simulink model "fivestatespace_revised"  (R2020a)
settings: Solver=VariableStepAuto  StartTime=0.0  StopTime=10.00  RelTol=1e-3
values from neighbouring files (symbols this model uses):
  alpha = (slope*pi)/180    (= 0)    [milestone2constants.m]
  Beq = 0.2963    [milestone2constants.m]
  Fd = 0    [milestone2constants.m]
  Jeq = 0.01802    [milestone2constants.m]
  Kb = 2.2179e-3    (= 0.0022179)    [milestone2constants.m]
  Keq = 0.74    [milestone2constants.m]
  Mg = M*g    (= 15.5979)    [milestone2constants.m]
  Mgmu = M*g*mu    (= 0)    [milestone2constants.m]
  r = 0.037    [milestone2constants.m]
  ra = 7.4    [milestone2constants.m]
  step_time = 10    [milestone2constants.m]
  theta_i = 0    [milestone2constants.m]
  threshold = 5    [milestone2constants.m]
  u_l_f = 9    [milestone2constants.m]
  u_l_i = 10    [milestone2constants.m]
  u_r_f = 3    [milestone2constants.m]
  u_r_i = 5    [milestone2constants.m]
  v_i = 0    [milestone2constants.m]
  v_txy = 0    [milestone2constants.m]
  v_w = 0    [milestone2constants.m]
  wl_i = 0    [milestone2constants.m]
  Wr = 0.18    [milestone2constants.m]
  wr_i = 0    [milestone2constants.m]
  x_i = 0    [milestone2constants.m]
  y_i = 0    [milestone2constants.m]
undefined symbols (not defined in the file or in its folder): k
settings Model: Creator=oliviaball  LastModifiedBy=oliviaball
settings DataIOCC: ReturnWorkspaceOutputs=off
settings DebuggingCC: ArithmeticOperatorsInVariantConditions=warning
settings SFSimCC: CustomCodeUndefinedFunction=UseInterfaceOnly

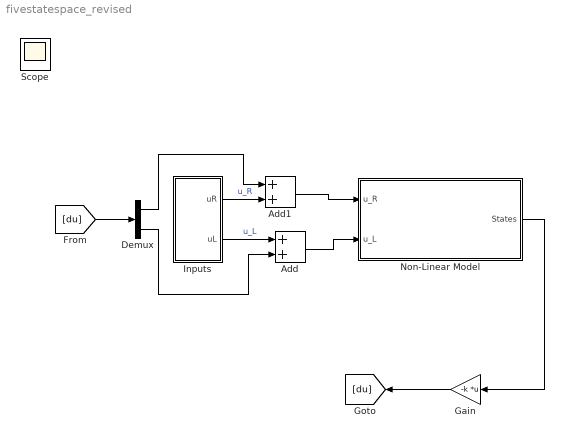
== system fivestatespace_revised ==
  Add : Sum
  Add1 : Sum
  Demux : Demux  Outputs=2
  Gain : Gain  Gain=-k  Multiplication=Matrix(K*u)
  Inputs : Subsystem
  Non-Linear Model : Subsystem
  Scope : Scope
  wires:
  Non-Linear Model/1(States) -> Gain/1
  Gain/1 -> [du]
  [du] -> Demux/1
  Inputs/2(uL) -> Add/1  "u_L"
  Add/1 -> Non-Linear Model/2(u_L)
  Demux/2 -> Add/2
  Inputs/1(uR) -> Add1/2  "u_R"
  Add1/1 -> Non-Linear Model/1(u_R)
  Demux/1 -> Add1/1

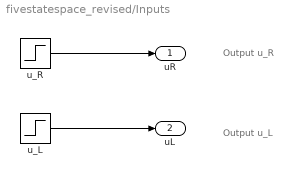
== system fivestatespace_revised/Inputs ==
  note: Output u_R
  note: Output u_L
  u_L : Step  Time=step_time  Before=u_l_i  After=u_l_f  SampleTime=0
  u_R : Step  Time=step_time  Before=u_r_i  After=u_r_f  SampleTime=0
  uR : Outport  VectorParamsAs1DForOutWhenUnconnected=off
  uL : Outport  Port=2  VectorParamsAs1DForOutWhenUnconnected=off
  wires:
  u_L/1 -> uL/1
  u_R/1 -> uR/1

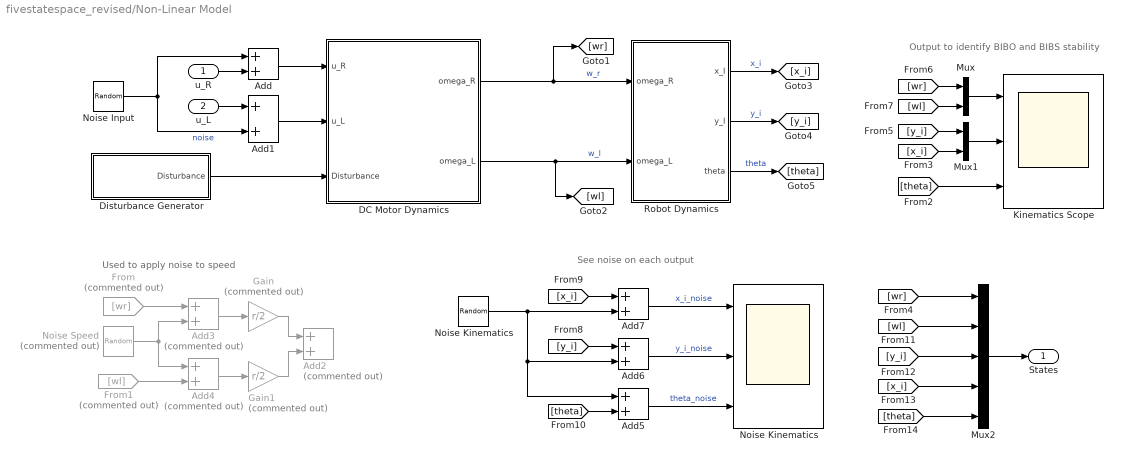
== system fivestatespace_revised/Non-Linear Model ==
  note: Used to apply noise to speed
  note: Output to identify BIBO and BIBS stability
  note: See noise on each output
  u_R : Inport
  u_L : Inport  Port=2
  Add{,1,5..7} (5 alike) : Sum
  Add2 : Sum  Commented=on
  Add3 : Sum  Commented=on
  Add4 : Sum  Commented=on
  DC Motor Dynamics : Subsystem
  "Disturbance Generator " : Subsystem
  From : From  Commented=on  GotoTag=wr
  From1 : From  Commented=on  GotoTag=wl
  Gain : Gain  Commented=on  Gain=r/2
  Gain1 : Gain  Commented=on  Gain=r/2
  Kinematics Scope : Scope  NumInputPorts=3
  Mux : Mux  Inputs=2
  Mux1 : Mux  Inputs=2
  Mux2 : Mux  Inputs=5
  "Noise Input " : RandomNumber  Variance=v_i  SampleTime=0.1
  Noise Kinematics : Scope  NumInputPorts=3
  "Noise Kinematics " : RandomNumber  Variance=v_txy  SampleTime=0.1
  Noise Speed : RandomNumber  Commented=on  Variance=v_w  SampleTime=0.1
  Robot Dynamics : Subsystem
  States : Outport
  wires:
  Robot Dynamics/2("y_I ") -> [y_i]  "y_i"
  DC Motor Dynamics/2(omega_L) -> Robot Dynamics/2(omega_L), [wl]  "w_l"
  DC Motor Dynamics/1(omega_R) -> Robot Dynamics/1(omega_R), [wr]  "w_r"
  Robot Dynamics/1(x_I) -> [x_i]  "x_i"
  u_R/1 -> Add/2
  Gain1/1 -> Add2/2
  Gain/1 -> Add2/1
  "Disturbance Generator "/1("Disturbance ") -> DC Motor Dynamics/3(Disturbance)
  Add/1 -> DC Motor Dynamics/1(u_R)
  Add1/1 -> DC Motor Dynamics/2(u_L)
  u_L/1 -> Add1/1
  "Noise Input "/1 -> Add/1, Add1/2  "noise"
  Add4/1 -> Gain1/1
  Add3/1 -> Gain/1
  Noise Speed/1 -> Add4/1, Add3/2
  "Noise Kinematics "/1 -> Add5/1, Add6/2, Add7/2
  Add7/1 -> Noise Kinematics/1  "x_i_noise"
  Add6/1 -> Noise Kinematics/2  "y_i_noise"
  Add5/1 -> Noise Kinematics/3  "theta_noise"
  Robot Dynamics/3(theta) -> [theta]  "theta"
  From/1 -> Add3/1
  From1/1 -> Add4/2
  Mux1/1 -> Kinematics Scope/2
  Mux/1 -> Kinematics Scope/1
  [x_i] -> Mux1/2
  [theta] -> Kinematics Scope/3
  [y_i] -> Mux1/1
  [wr] -> Mux/1
  [wl] -> Mux/2
  [y_i] -> Add6/1
  [x_i] -> Add7/1
  [theta] -> Add5/2
  Mux2/1 -> States/1
  [wr] -> Mux2/1
  [wl] -> Mux2/2
  [y_i] -> Mux2/3
  [x_i] -> Mux2/4
  [theta] -> Mux2/5

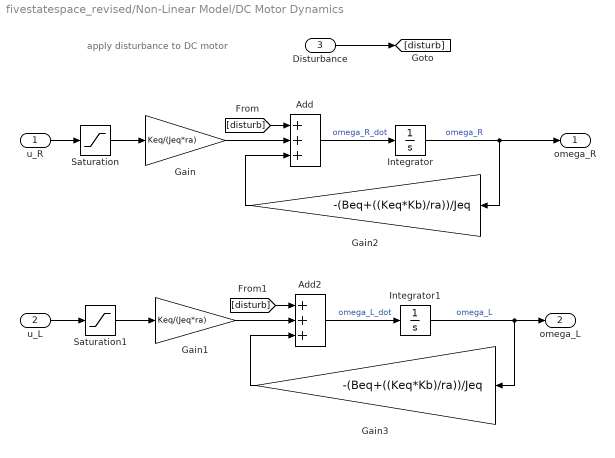
== system fivestatespace_revised/Non-Linear Model/DC Motor Dynamics ==
  note: apply disturbance to DC motor
  u_R : Inport
  u_L : Inport  Port=2
  Disturbance : Inport  Port=3
  Add : Sum  Inputs=+++
  Add2 : Sum  Inputs=+++
  Gain : Gain  Gain=Keq/(Jeq*ra)
  Gain1 : Gain  Gain=Keq/(Jeq*ra)
  Gain2 : Gain  Gain=-(Beq+((Keq*Kb)/ra))/Jeq
  Gain3 : Gain  Gain=-(Beq+((Keq*Kb)/ra))/Jeq
  Integrator : Integrator  InitialCondition=wr_i
  Integrator1 : Integrator  InitialCondition=wl_i
  Saturation : Saturate  UpperLimit=10  LowerLimit=-10
  Saturation1 : Saturate  UpperLimit=10  LowerLimit=-10
  omega_R : Outport  VectorParamsAs1DForOutWhenUnconnected=off
  omega_L : Outport  Port=2  VectorParamsAs1DForOutWhenUnconnected=off
  wires:
  Add/1 -> Integrator/1  "omega_R_dot"
  Integrator/1 -> omega_R/1, Gain2/1  "omega_R"
  Add2/1 -> Integrator1/1  "omega_L_dot"
  Integrator1/1 -> omega_L/1, Gain3/1  "omega_L"
  Gain3/1 -> Add2/3
  Gain1/1 -> Add2/2
  Gain2/1 -> Add/3
  Gain/1 -> Add/2
  [disturb] -> Add/1
  Disturbance/1 -> [disturb]
  [disturb] -> Add2/1
  u_R/1 -> Saturation/1
  Saturation/1 -> Gain/1
  u_L/1 -> Saturation1/1
  Saturation1/1 -> Gain1/1

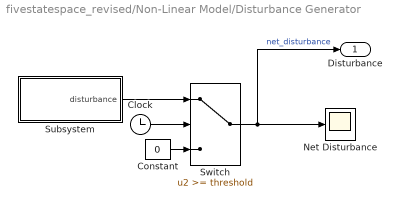
== system fivestatespace_revised/Non-Linear Model/Disturbance Generator  ==
  Clock : Clock
  Constant : Constant  Value=0
  "Net Disturbance " : Scope
  Subsystem : Subsystem
  Switch : Switch  Threshold=threshold
  "Disturbance " : Outport  VectorParamsAs1DForOutWhenUnconnected=off
  wires:
  Clock/1 -> Switch/2
  Constant/1 -> Switch/3
  Switch/1 -> "Disturbance "/1, "Net Disturbance "/1  "net_disturbance"
  Subsystem/1(disturbance) -> Switch/1

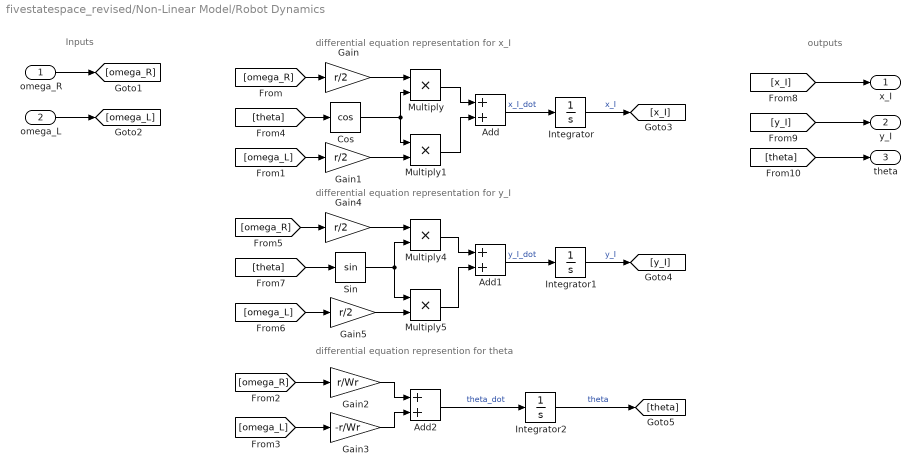
== system fivestatespace_revised/Non-Linear Model/Robot Dynamics ==
  note: Inputs
  note: outputs
  note: differential equation representation for y_I
  note: differential equation represention for theta
  note: differential equation representation for x_I
  omega_R : Inport
  omega_L : Inport  Port=2
  Add : Sum
  Add1 : Sum
  Add2 : Sum
  Cos : Trigonometry  Operator=cos
  Gain{,1,4..5} (4 alike) : Gain  Gain=r/2
  Gain2 : Gain  Gain=r/Wr
  Gain3 : Gain  Gain=-r/Wr
  Integrator : Integrator  InitialCondition=x_i
  Integrator1 : Integrator  InitialCondition=y_i
  Integrator2 : Integrator  InitialCondition=theta_i
  Multiply{,1,4..5} (4 alike) : Product
  Sin : Trigonometry
  x_I : Outport  VectorParamsAs1DForOutWhenUnconnected=off
  "y_I " : Outport  Port=2  VectorParamsAs1DForOutWhenUnconnected=off
  theta : Outport  Port=3  VectorParamsAs1DForOutWhenUnconnected=off
  wires:
  omega_R/1 -> [omega_R]
  omega_L/1 -> [omega_L]
  [omega_L] -> Gain5/1
  Multiply5/1 -> Add1/2
  [omega_R] -> Gain4/1
  Integrator/1 -> [x_I]  "x_I"
  [theta] -> theta/1
  Gain/1 -> Multiply/1
  Integrator1/1 -> [y_I]  "y_I"
  Multiply4/1 -> Add1/1
  Add2/1 -> Integrator2/1  "theta_dot"
  Add1/1 -> Integrator1/1  "y_I_dot"
  Multiply1/1 -> Add/2
  Gain4/1 -> Multiply4/1
  Multiply/1 -> Add/1
  Gain2/1 -> Add2/1
  [y_I] -> "y_I "/1
  [x_I] -> x_I/1
  Gain5/1 -> Multiply5/2
  [omega_L] -> Gain1/1
  [theta] -> Cos/1
  Gain1/1 -> Multiply1/2
  [theta] -> Sin/1
  [omega_L] -> Gain3/1
  Add/1 -> Integrator/1  "x_I_dot"
  Sin/1 -> Multiply5/1, Multiply4/2
  Integrator2/1 -> [theta]  "theta"
  [omega_R] -> Gain/1
  Cos/1 -> Multiply1/1, Multiply/2
  [omega_R] -> Gain2/1
  Gain3/1 -> Add2/2

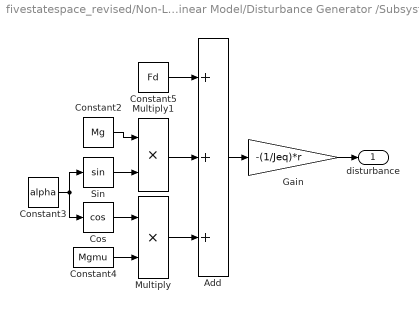
== system fivestatespace_revised/Non-Linear Model/Disturbance Generator /Subsystem ==
  Add : Sum  Inputs=+++
  Constant2 : Constant  Value=Mg
  Constant3 : Constant  Value=alpha
  Constant4 : Constant  Value=Mgmu
  Constant5 : Constant  Value=Fd
  Cos : Trigonometry  Operator=cos
  Gain : Gain  Gain=-(1/Jeq)*r
  Multiply : Product
  Multiply1 : Product
  Sin : Trigonometry
  disturbance : Outport  VectorParamsAs1DForOutWhenUnconnected=off
  wires:
  Constant3/1 -> Sin/1, Cos/1
  Constant4/1 -> Multiply/2
  Cos/1 -> Multiply/1
  Sin/1 -> Multiply1/2
  Constant2/1 -> Multiply1/1
  Constant5/1 -> Add/1
  Multiply1/1 -> Add/2
  Multiply/1 -> Add/3
  Add/1 -> Gain/1
  Gain/1 -> disturbance/1
